simulink model "even_four_bitparitygenerator"  (R2021b)
settings: Solver=VariableStepAuto  StartTime=0.0  StopTime=.2  RelTol=1e-3
settings Model: Creator=Joshua  LastModifiedBy=Joshua

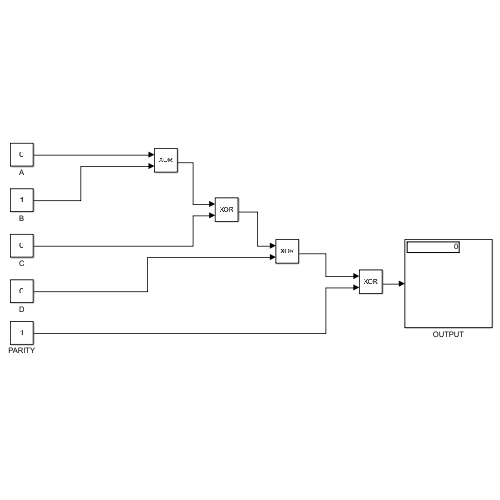
[thumbnail: Simulink's stored preview of the top-level diagram]
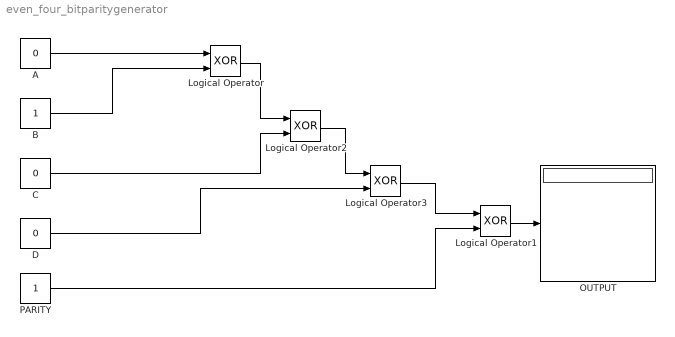
== system even_four_bitparitygenerator ==
  A : Constant  Value=0
  B : Constant
  C : Constant  Value=0
  D : Constant  Value=0
  Logical Operator{,1..3} (4 alike) : Logic  Operator=XOR  AllPortsSameDT=off  OutDataTypeStr=boolean
  OUTPUT : Display
  PARITY : Constant
  wires:
  A/1 -> Logical Operator/1
  B/1 -> Logical Operator/2
  C/1 -> Logical Operator2/2
  Logical Operator/1 -> Logical Operator2/1
  Logical Operator2/1 -> Logical Operator3/1
  D/1 -> Logical Operator3/2
  PARITY/1 -> Logical Operator1/2
  Logical Operator3/1 -> Logical Operator1/1
  Logical Operator1/1 -> OUTPUT/1
